simulink model "ADSBSimulinkExample"  (R2024b)
settings: Solver=FixedStepDiscrete  StartTime=0.0  StopTime=10  RelTol=1e-3
PreLoadFcn:
  | radioSampleRate = 2.4e6;
  | adsbParam = helperAdsbConfig(radioSampleRate);
  | load dataAdsbBusObjects
  | LaunchMap = 0;
  | LogData = 0;
PostLoadFcn:
  | if exist('sdruroot', 'file')
  |     sdruExampleSetAvailableRadio();
  |     if (strcmp(get_param([gcs '/Signal Source Selector'],'OverrideUsingVariant'),'V_4'))
  |        radioSampleRate = 20e6;
  |        platform = get_param([gcs '/SDRu Receiver'], 'Platform');
  |        adsbParam = helperAdsbConfig(platform);
  |     end
  | end
InitFcn:
  | load dataAdsbBusObjects
  | if (strcmp(get_param([gcs '/Signal Source Selector'],'OverrideUsingVariant'),'V_4'))
  |     radioSampleRate = 20e6;
  |     platform = get_param([gcs '/SDRu Receiver'], 'Platform');
  |     adsbParam = helperAdsbConfig(platform);
  |     helperAdsbCheckModelParams(platform);
  |     switch platform
  |       case 'X300'
  |         set_param([gcs,'/SDRu Receiver'], 'masterClkRateX300','200e6');
  |       case 'X310'
  |         set_param([gcs,'/SDRu Receiver'], 'masterClkRateX310','200e6');
  |       case 'N300'
  |         set_param([gcs,'/SDRu Receiver'], 'masterClkRateN300','153.6e6');
  |       case 'N310'
  |         set_param([gcs,'/SDRu Receiver'], 'masterClkRateN310','153.6e6');
  |       case 'N320/N321'
  |          set_param([gcs,'/SDRu Receiver'], 'masterClkRateN320','200e6');
  |       case 'N200/N210/USRP2'
  |          set_param([gcs,'/SDRu Receiver'], 'masterClkRateN320','200e6');
  |     end
  |     clear platform
  | else
  |     adsbParam = helperAdsbConfig;
  |     helperAdsbCheckModelParams;
  | end
undefined symbols (not defined in the file or in its folder): Fs, ip, usb
libraries: simulink x2, ADSBExampleLib x2, plutoradiolib x1, commsource2 x1, sdrrlib x1, commsdrhw_v2 x1
CloseFcn:
  | hFig = findall(0, 'Type', 'figure', 'Tag', 'ADS-B Aircraft Tracking');
  | if ishghandle(hFig)
  | close(hFig);
  | end
  | clear hFig
settings Model: Creator=The MathWorks, Inc.  LastModifiedBy=samue
settings SolverCC: AlgebraicLoopSolver=TrustRegion  AutoInsertRateTranBlk=on
settings DataIOCC: LimitDataPoints=on  SaveFormat=Array  SaveOutput=off  SaveTime=off  ReturnWorkspaceOutputs=off
settings OptimizationCC: BooleanDataType=off  DefaultParameterBehavior=Inlined  ReuseModelBlockBuffer=off  LocalBlockOutputs=off  LifeSpan=inf
settings DebuggingCC: AlgebraicLoopMsg=error  SingleTaskRateTransMsg=warning  ParameterPrecisionLossMsg=none  UnconnectedInputMsg=warning  UnconnectedOutputMsg=warning  UnconnectedLineMsg=warning  AllowSymbolicDim=off  SFUnexpectedBacktrackingDiag=warning  SFNoUnconditionalDefaultTransitionDiag=warning  SFExecutionAtInitializationDiag=none  ArithmeticOperatorsInVariantConditions=warning
settings ModelReferenceCC: EnableRefExpFcnMdlSchedulingChecks=on  PropagateSignalLabelsOutOfModel=off
settings SFSimCC: SimUseLocalCustomCode=off  CustomCodeUndefinedFunction=UseInterfaceOnly
settings RTWCC: RTWUseLocalCustomCode=off  GPUComputeCapability=3.5  DLArmComputeVersion=19.05
settings CodeAppCC: StateflowObjectComments=on
settings GRTTargetCC: TargetLangStandard=C89/C90 (ANSI)
settings ConfigComp: CovScope=ReferencedModels  CovMetricSettings=dw  CovSaveCumulativeToWorkspaceVar=on  CovSaveSingleToWorkspaceVar=on  CovExternalEMLEnable=off  CovSFcnEnable=off

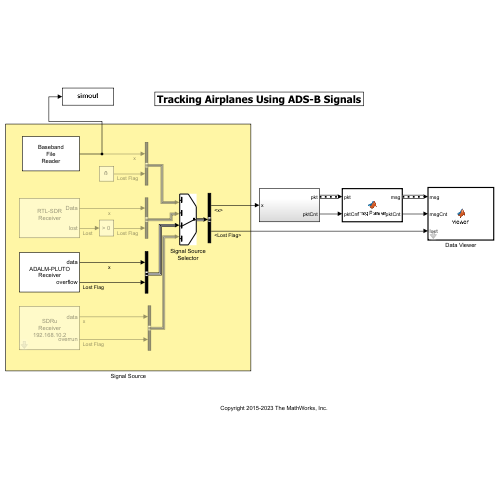
[thumbnail: Simulink's stored preview of the top-level diagram]
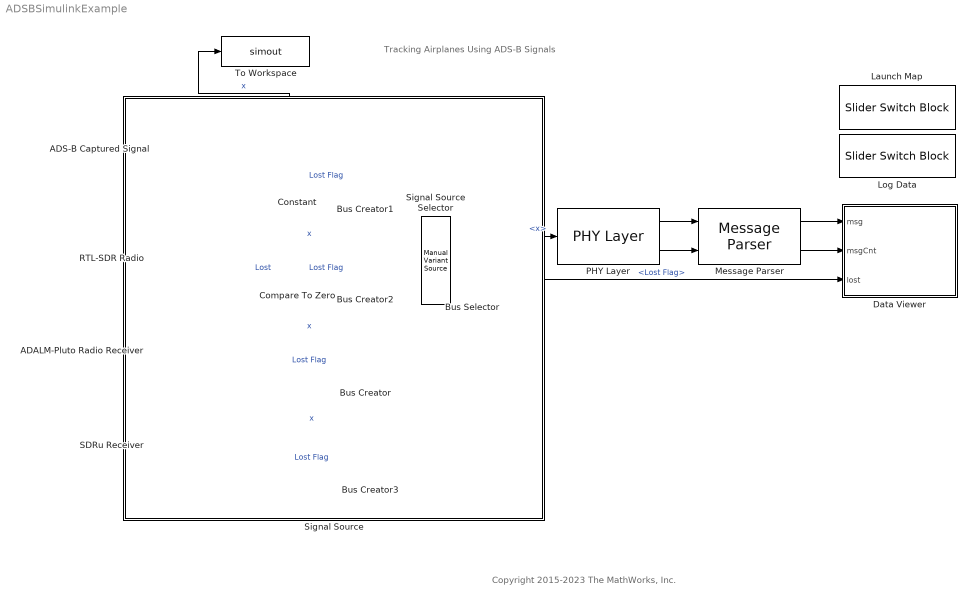
== system ADSBSimulinkExample ==
  note: Tracking Airplanes Using ADS-B Signals
  note: Copyright 2015-2023 The MathWorks, Inc.
  ADALM-Pluto Radio Receiver : plutoradiolib/ADALM-Pluto Radio Receiver  RadioID=usb:0  uri=ip:10.0.0.200  CenterFrequencySource=Dialog  CenterFrequency=1090e6  GainSource=AGC Slow Attack  GainSourceBlock=AGC Slow Attack  Gain=10  ChannelMapping=1  BasebandSampleRate=adsbParam.FrontEndSampleRate  OutputDataType=single  SamplesPerFrame=adsbParam.SamplesPerFrame  OverflowOutputPort=on  EnableBurstMode=off  NumFramesInBurst=1  ShowAdvancedProperties=off  UseCustomFilter=off  filtPathRates=[ 737280000, 11520000, 3840000, 1920000, 960000, 240000 ]  filtCoefficients=round( fir1( 127, 0.75 )*2^15*10^1.2 )  filtCoefficientSize=128  filtDecimInterpFactor=4  filtGain=-12  filtRFBandwidth=18e6  filterConfigStruct=struct()  EnableQuadratureCorrection=on  EnableRFDCCorrection=on  EnableBasebandDCCorrection=on  FrequencyCorrection=0  OverrideSampleTime=off  SampleTime=0.02  DataTimeout=Inf  ENSMPinControlMode=None  BISTLoopbackMode=Disabled  BISTToneInject=Disabled  BISTSignalGen=PRBS  BISTToneFreq=Fs/32  BISTToneLevel=0
  ADS-B Captured Signal : commsource2/Baseband File Reader  Filename=adsb_capture_01.bb  InheritSampleTimeFromFile=on  SampleTime=1  SamplesPerFrame=adsbParam.SamplesPerFrame  CyclicRepetition=on  FileEndOutputPort=off  SimulateUsing=Code generation
  Bus Creator{,1..3} (4 alike) : BusCreator  Inputs=2
  Bus Selector : BusSelector  OutputSignals=x,Lost Flag
  Compare To Zero : simulink/Logic and Bit Operations/Compare To Zero  relop=>  OutDataTypeStr=boolean
  Constant : Constant  Value=0
  Data Viewer : MATLAB Function  StopFcn=|  TreatAsAtomicUnit=on  mask(ADS-B viewer){logfilename=adsb_messages.txt}
      | adsbGUI=findall(0,'type','figure','Tag','ADS-B Aircraft Tracking');
      | if ~isempty(adsbGUI)
      |   viewer=getappdata(adsbGUI,'ViewerHandle');
      |   stop(viewer);
      | end
      mask prompts: logfilename "Log data to file :"
  Launch Map : SliderSwitchBlock
      settings: Values={{'Off', 'On'}, [0 1]}
  Log Data : SliderSwitchBlock
      settings: Values={{'Off', 'On'}, [0 1]}
  Message Parser : ADSBExampleLib/Message Parser  SystemSampleTime=-1  VariantActivationTime=update diagram  AllowFlexibleInterface=on  Latency=0  AutoFrameSizeCalculation=off
  PHY Layer : ADSBExampleLib/PHY Layer  SystemSampleTime=-1  VariantActivationTime=update diagram  AllowFlexibleInterface=on  Latency=0  AutoFrameSizeCalculation=off
  RTL-SDR Radio : sdrrlib/RTL-SDR Receiver  IPAddress=0  CenterFrequencySource=Dialog  CenterFrequency=1090e6  GainSource=Dialog  Gain=60  ADCRate=adsbParam.FrontEndSampleRate  FrequencyCorrection=0  LostSamplesOutputPort=on  LatencyOutputPort=off  OutputDataType=single  FrameLength=adsbParam.SamplesPerFrame  EnableBurstMode=off  NumFramesInBurst=100  sobjType=sdrr.internal.SDRRTLReceiverSL  dataUDPPort=-1  ctrlUDPPort=-1  subDeviceList=nosubdev  sdrBlockType=SDRBlockTypeSLT.SDRRxBlock  requester=UNUSED_BY_SFCN  sdrExecutionMode=SDRExecutionModeSLT.ExecModeHW  BypassUserLogic=off  DecimatorSelect=DDC decimator  SourceSelect=RF data  SineAmplitude=16000  EnableInternalClock=off  BypassIQBalance=off  IFBandwidth=40e6  ADCRateSource=Dialog  IntermediateFrequency=0  DecimationFactorSource=Dialog  DecimationFactor=512  RFFrequencyIsTunable=logical(0)  SampleTime=(adsbParam.SamplesPerFrame)/(adsbParam.FrontEndSampleRate)  IFBandwidthSource=Dialog  SineFrequency=30000  BypassDCBlockingFilter=off  IntermediateFrequencySource=Dialog  IQBalanceCoefficients=64  SkipAllHardwareResetAndInitialization=off  EnableIQCalibrationTable=on  CacheIQCalibrationTable=off  EnableOffsetTuning=off  EnableRTLAGC=off  EnableTestMode=off  EnableTunerAGC=off  FrequencyCorrectionSource=Dialog  NumMLBuffers=128  NumUSBBuffers=16  RTLCrystalFrequency=28800000  TunerCrystalFrequency=28800000
  SDRu Receiver : commsdrhw_v2/SDRu Receiver  rxtx=rx  initializeIPAddress=0  devMap=10  USRP2_IP=192.168.10.2  USRP_IP_X300=192.168.10.2  USRP_IP_X310=192.168.70.2  USRP_IP_N300=192.168.10.2  USRP_IP_N310=192.168.10.2  USRP_IP_N320=192.168.10.2  USRP_serialNumB200=30EA06C  USRP_serialNumB210=3136D21  platform=N200/N210/USRP2  prevPlatform=N200/N210/USRP2  lastIPAddressPopup=192.168.10.2  USRP_ID=192.168.10.2  LastIPAddress=192.168.10.2  IsTwinRXDaughterboard=off  EnableTwinRXPhaseSync=off  losrc=0  ChannelMapping=1  centerFrequencySrc=Dialog  centerFrequency=1090e6  loOffsetSrc=Dialog  loOffset=0  gainSrc=Dialog  gain=adsbParam.Gain  PPSSource=Internal  clockSource=Internal  EnableGPSLock=off  EnsureSyncGPSTime=off  EnableTimeTrigger=off  triggerTime=5  enableMIMOCableSync=off  EnableRefLock=off  masterClkRateParam=100e6  masterClkRateB200=adsbParam.MasterClockRate  masterClkRateB210=adsbParam.MasterClockRate  masterClkRateX300=200e6  masterClkRateX310=200e6  masterClkRateN300=153.6e6  masterClkRateN310=153.6e6  masterClkRateN320=200e6  masterClkRate=100e6  masterClkRateTwinRX=200e6  decimInterpSrc=Dialog  decimInterpPort=512  lastDecimSource=Dialog  decimInterp=adsbParam.DecimationFactor  USRP2_IP_NUM=[49 57 50 46 49 54 56 46 49 48 46 50]  sampleRate=20000000  sampleTime=(5)/100000000  TransportDataType=int16  overrunUnderrunPort=on  dataLengthPort=off  EnableTimeStamps=off  outputDatatype=single  frameLength=51840  HOST_DATA_PORT=0  HOST_CONTROL_PORT=0  USRP2_DATA_PORT=0  USRP2_CONTROL_PORT=0  bufferMode=Continuous streaming  EnableBurstMode=off  NumFramesInBurst=100
      settings: SourceProductName=Communications Toolbox Support Package for USRP(TM) Radio
  Signal Source : Subsystem
      mask Display: disp('')
  Signal Source Selector : simulink/Signal Routing/Manual Variant Source  NumChoices=4  LabelModeActiveChoice=V_3
  To Workspace : ToWorkspace  VariableName=simout  SaveFormat=Timeseries  SampleTime=-1
  wires:
  Message Parser/1 -> Data Viewer/1(msg)
  Message Parser/2 -> Data Viewer/2(msgCnt)
  PHY Layer/1 -> Message Parser/1
  PHY Layer/2 -> Message Parser/2
  Bus Selector/2 -> Data Viewer/3(lost)  "<Lost Flag>"
  Bus Selector/1 -> PHY Layer/1  "<x>"
  RTL-SDR Radio/1 -> Bus Creator2/1  "x"
  ADS-B Captured Signal/1 -> To Workspace/1, Bus Creator1/1  "x"
  Bus Creator2/1 -> Signal Source Selector/2
  ADALM-Pluto Radio Receiver/1 -> Bus Creator/1  "x"
  Signal Source Selector/1 -> Bus Selector/1
  Bus Creator/1 -> Signal Source Selector/3
  Bus Creator1/1 -> Signal Source Selector/1
  RTL-SDR Radio/2 -> Compare To Zero/1  "Lost"
  Compare To Zero/1 -> Bus Creator2/2  "Lost Flag"
  Constant/1 -> Bus Creator1/2  "Lost Flag"
  ADALM-Pluto Radio Receiver/2 -> Bus Creator/2  "Lost Flag"
  SDRu Receiver/2 -> Bus Creator3/2  "Lost Flag"
  SDRu Receiver/1 -> Bus Creator3/1  "x"
  Bus Creator3/1 -> Signal Source Selector/4

== system ADSBSimulinkExample/Signal Source ==

== matlab function ADSBSimulinkExample/Data Viewer ==
  data: msg input; msgCnt input; lost input; LaunchMap parameter; LogData parameter
function viewer(msg, msgCnt, lost, LaunchMap, LogData)
%#codegen

persistent resetGUI

if isempty(resetGUI)
  resetGUI = true;
end

block = 'ADSBSimulinkExample/Data Viewer';

coder.extrinsic('helperAdsbViewerAdaptor');

coder.extrinsic('get_param','set_param');

Logfilename = get_param(block,'logfilename');

helperAdsbViewerAdaptor(msg, msgCnt, resetGUI, LaunchMap, LogData, Logfilename, lost);

resetGUI = false;
